simulink subsystem "SystemControl"  (R2019b)
settings: Solver=VariableStepAuto  StartTime=0.0  StopTime=10.0  RelTol=1e-3
libraries: FunctionCallDivider x2
settings Model: Creator=Nick  LastModifiedBy=Nick

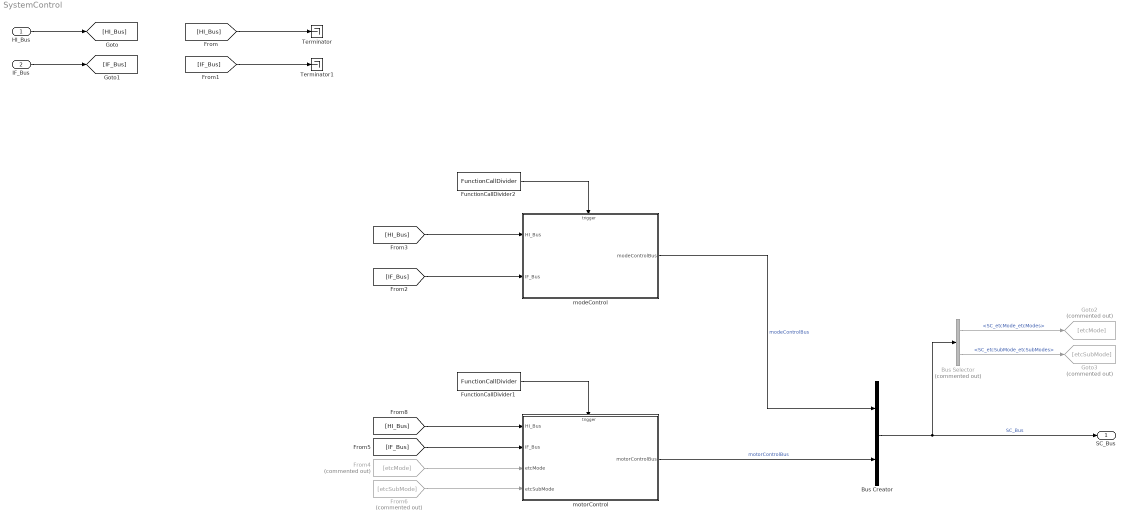
== system SystemControl ==
  HI_Bus : Inport
  IF_Bus : Inport  Port=2
  Bus Creator : BusCreator  Inputs=2
  Bus Selector : BusSelector  Commented=on  OutputSignals=modeControlBus.SC_etcMode_etcModes,modeControlBus.SC_etcSubMode_etcSubModes
  From4 : From  Commented=on  GotoTag=etcMode
  From6 : From  Commented=on  GotoTag=etcSubMode
  FunctionCallDivider1 : FunctionCallDivider/Algroithms/FunctionCallDivider  counts=1
  FunctionCallDivider2 : FunctionCallDivider/Algroithms/FunctionCallDivider  counts=10
  Goto2 : Goto  Commented=on  GotoTag=etcMode
  Goto3 : Goto  Commented=on  GotoTag=etcSubMode
  Terminator : Terminator
  Terminator1 : Terminator
  modeControl : Subsystem  TreatAsAtomicUnit=on
  motorControl : Subsystem  TreatAsAtomicUnit=on
  SC_Bus : Outport
  wires:
  IF_Bus/1 -> [IF_Bus]
  Bus Creator/1 -> SC_Bus/1, Bus Selector/1  "SC_Bus"
  [HI_Bus] -> Terminator/1
  [IF_Bus] -> Terminator1/1
  HI_Bus/1 -> [HI_Bus]
  [HI_Bus] -> motorControl/1(HI_Bus)
  FunctionCallDivider1/1 -> motorControl/Trigger
  [IF_Bus] -> motorControl/2(IF_Bus)
  motorControl/1(motorControlBus) -> Bus Creator/2  "motorControlBus"
  [IF_Bus] -> modeControl/2(IF_Bus)
  FunctionCallDivider2/1 -> modeControl/Trigger
  [HI_Bus] -> modeControl/1(HI_Bus)
  modeControl/1(modeControlBus) -> Bus Creator/1  "modeControlBus"
  Bus Selector/1 -> Goto2/1  "<SC_etcMode_etcModes>"
  From4/1 -> motorControl/3(etcMode)
  Bus Selector/2 -> Goto3/1  "<SC_etcSubMode_etcSubModes>"
  From6/1 -> motorControl/4(etcSubMode)

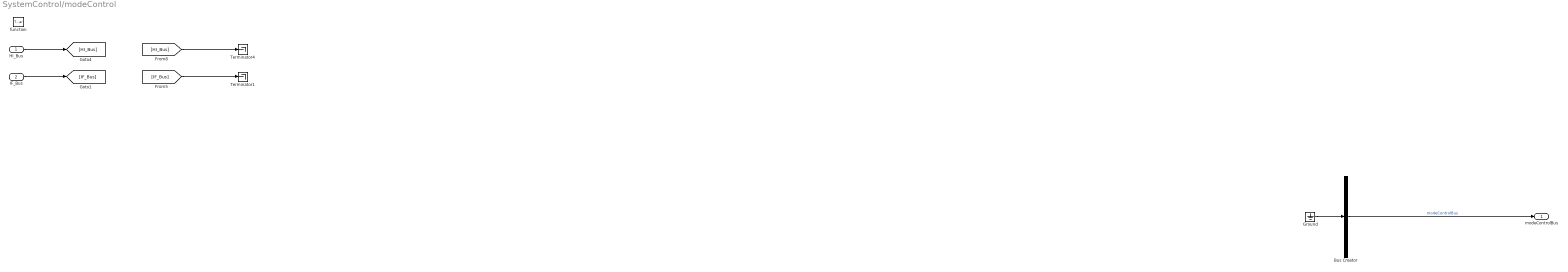
== system SystemControl/modeControl ==
  HI_Bus : Inport
  IF_Bus : Inport  Port=2
  function : TriggerPort  TriggerType=function-call  VariantControl=Variant
  Bus Creator : BusCreator  Inputs=1
  Ground : Ground
  Terminator1 : Terminator
  Terminator4 : Terminator
  modeControlBus : Outport
  wires:
  Ground/1 -> Bus Creator/1
  Bus Creator/1 -> modeControlBus/1  "modeControlBus"
  [IF_Bus] -> Terminator1/1
  HI_Bus/1 -> [HI_Bus]
  [HI_Bus] -> Terminator4/1
  IF_Bus/1 -> [IF_Bus]

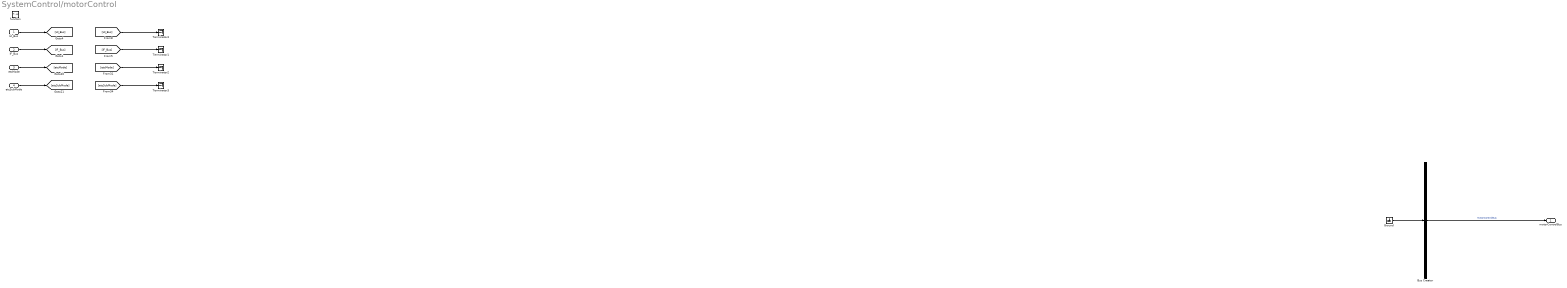
== system SystemControl/motorControl ==
  HI_Bus : Inport
  IF_Bus : Inport  Port=2
  etcMode : Inport  Port=3
  etcSubMode : Inport  Port=4
  function : TriggerPort  TriggerType=function-call  VariantControl=Variant
  Bus Creator : BusCreator  Inputs=1
  Ground : Ground
  Terminator{1..4} (4 alike) : Terminator
  motorControlBus : Outport
  wires:
  Ground/1 -> Bus Creator/1
  [etcSubMode] -> Terminator3/1
  etcSubMode/1 -> [etcSubMode]
  [etcMode] -> Terminator2/1
  etcMode/1 -> [etcMode]
  Bus Creator/1 -> motorControlBus/1  "motorControlBus"
  [IF_Bus] -> Terminator1/1
  HI_Bus/1 -> [HI_Bus]
  [HI_Bus] -> Terminator4/1
  IF_Bus/1 -> [IF_Bus]
